simulink model "block_model2018a"  (R2018a)
settings: Solver=VariableStepAuto  StartTime=0.0  StopTime=80  RelTol=1e-3
undefined symbols (not defined in the file or in its folder): DiscIntNeverNeededParam
libraries: simulink x4
settings Model: Creator=igorbeduin  LastModifiedBy=igorbeduin
settings DataIOCC: ReturnWorkspaceOutputs=on
settings SFSimCC: SimUseLocalCustomCode=on
settings RTWCC: RTWUseLocalCustomCode=on

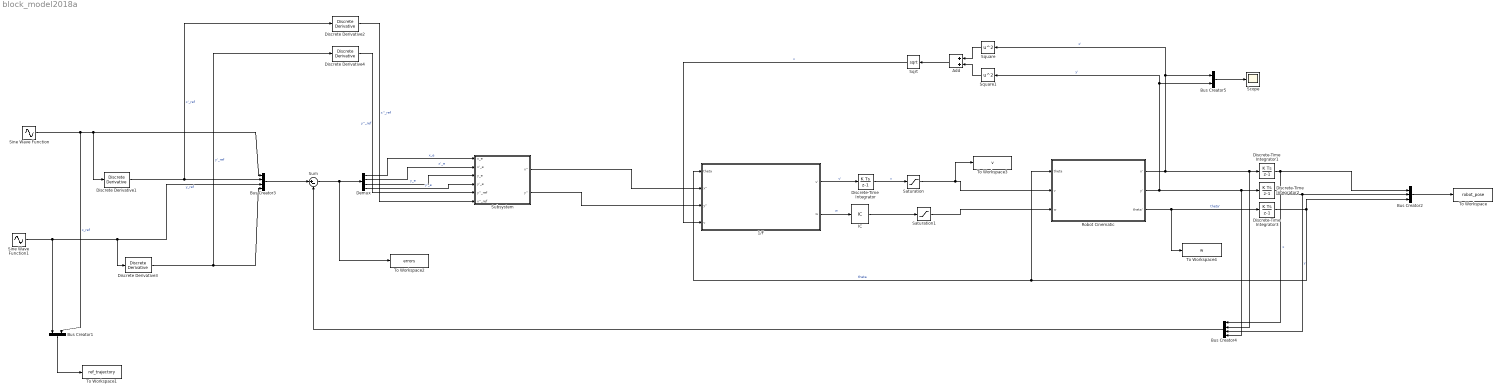
== system block_model2018a ==
  1/F : Subsystem
  Add : Sum
  Bus Creator1 : BusCreator  Inputs=2
  Bus Creator2 : BusCreator  Inputs=3
  Bus Creator3 : BusCreator  Inputs=4
  Bus Creator4 : BusCreator  Inputs=4
  Bus Creator5 : BusCreator  Inputs=2
  Demux : Demux
  Discrete Derivative{1..4} (4 alike) : simulink/Discrete/Discrete Derivative  gainval=1.0  ICPrevScaledInput=0  OutMin=[]  OutMax=[]  OutDataType=fixdt(1, 16)  OutScaling=2^-10  DoSatur=off
  Discrete-Time Integrator : DiscreteIntegrator  SampleTime=0.016  ICPrevOutput=DiscIntNeverNeededParam  ICPrevScaledInput=DiscIntNeverNeededParam
  Discrete-Time Integrator1 : DiscreteIntegrator  InitialCondition=0.5  SampleTime=-1  ICPrevOutput=DiscIntNeverNeededParam  ICPrevScaledInput=DiscIntNeverNeededParam
  Discrete-Time Integrator2 : DiscreteIntegrator  InitialCondition=-0.5  SampleTime=-1  ICPrevOutput=DiscIntNeverNeededParam  ICPrevScaledInput=DiscIntNeverNeededParam
  Discrete-Time Integrator3 : DiscreteIntegrator  SampleTime=-1  ICPrevOutput=DiscIntNeverNeededParam  ICPrevScaledInput=DiscIntNeverNeededParam
  IC : InitialCondition  Value=0
  Robot Cinematic : Subsystem
  Saturation : Saturate  UpperLimit=1.2  LowerLimit=-1.2
  Saturation1 : Saturate  UpperLimit=40  LowerLimit=-40
  Scope : Scope
  Sine Wave Function : Sin  Frequency=2*pi/30  SampleTime=0.016
  Sine Wave Function1 : Sin  Frequency=2*2*pi/30  SampleTime=0.016
  Sqrt : Sqrt  SaturateOnIntegerOverflow=on
  Square : Math  Operator=square  SaturateOnIntegerOverflow=on
  Square1 : Math  Operator=square  SaturateOnIntegerOverflow=on
  Subsystem : Subsystem
  Sum : Sum  Inputs=|+-
  To Workspace : ToWorkspace  VariableName=robot_pose  SaveFormat=Timeseries  SampleTime=-1
  To Workspace1 : ToWorkspace  VariableName=ref_trajectory  SaveFormat=Timeseries  SampleTime=-1
  To Workspace2 : ToWorkspace  VariableName=errors  SaveFormat=Timeseries  SampleTime=-1
  To Workspace3 : ToWorkspace  VariableName=v  SaveFormat=Timeseries  SampleTime=-1
  To Workspace4 : ToWorkspace  VariableName=w  SaveFormat=Timeseries  SampleTime=-1
  wires:
  Robot Cinematic/1(x') -> Bus Creator4/2, Discrete-Time Integrator1/1, Square/1, Bus Creator5/1  "x'"
  Robot Cinematic/2(y') -> Bus Creator4/4, Discrete-Time Integrator2/1, Bus Creator5/2, Square1/1  "y'"
  Robot Cinematic/3(theta') -> To Workspace4/1, Discrete-Time Integrator3/1  "theta'"
  1/F/1(v') -> Discrete-Time Integrator/1  "v'"
  1/F/2(w) -> IC/1  "w"
  Discrete-Time Integrator1/1 -> Bus Creator2/1, Bus Creator4/1  "x"
  Discrete-Time Integrator2/1 -> Bus Creator2/2, Bus Creator4/3  "y"
  Discrete-Time Integrator3/1 -> Robot Cinematic/1(theta), 1/F/1(theta), Bus Creator2/3  "theta"
  Discrete Derivative1/1 -> Discrete Derivative2/1, Bus Creator3/2  "x'_ref"
  Discrete Derivative3/1 -> Bus Creator3/4, Discrete Derivative4/1  "y'_ref"
  Discrete Derivative2/1 -> Subsystem/6(x''_ref)  "x''_ref"
  Discrete Derivative4/1 -> Subsystem/5(y''_ref)  "y''_ref"
  Subsystem/1(x'') -> 1/F/2(x'')
  Subsystem/2(y'') -> 1/F/3(y'')
  Square/1 -> Add/1
  Square1/1 -> Add/2
  Add/1 -> Sqrt/1
  Sqrt/1 -> 1/F/4(v)  "v"
  Bus Creator2/1 -> To Workspace/1
  Bus Creator1/1 -> To Workspace1/1
  Bus Creator3/1 -> Sum/1
  Bus Creator4/1 -> Sum/2
  Sum/1 -> To Workspace2/1, Demux/1
  Demux/1 -> Subsystem/1(x_e)  "x_e"
  Demux/2 -> Subsystem/2(x'_e)  "x'_e"
  Demux/3 -> Subsystem/3(y_e)  "y_e"
  Demux/4 -> Subsystem/4(y'_e)  "y'_e"
  Discrete-Time Integrator/1 -> Saturation/1  "v"
  Bus Creator5/1 -> Scope/1
  Saturation/1 -> To Workspace3/1, Robot Cinematic/2(v)
  Saturation1/1 -> Robot Cinematic/3(w)
  IC/1 -> Saturation1/1
  Sine Wave Function/1 -> Bus Creator3/1, Discrete Derivative1/1, Bus Creator1/2  "x_ref"
  Sine Wave Function1/1 -> Bus Creator3/3, Discrete Derivative3/1, Bus Creator1/1  "y_ref"

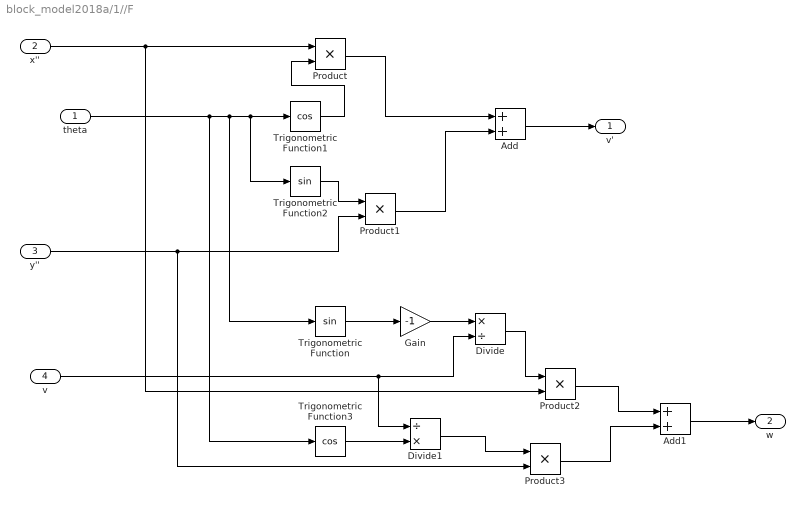
== system block_model2018a/1//F ==
  theta : Inport
  x'' : Inport  Port=2
  y'' : Inport  Port=3
  v : Inport  Port=4
  Add : Sum
  Add1 : Sum
  Divide : Product  Inputs=*/
  Divide1 : Product  Inputs=/*
  Gain : Gain  Gain=-1
  Product{,1..3} (4 alike) : Product
  Trigonometric Function : Trigonometry
  Trigonometric Function1 : Trigonometry  Operator=cos
  Trigonometric Function2 : Trigonometry
  Trigonometric Function3 : Trigonometry  Operator=cos
  v' : Outport
  w : Outport  Port=2
  wires:
  x''/1 -> Product2/2, Product/1
  theta/1 -> Trigonometric Function/1, Trigonometric Function2/1, Trigonometric Function1/1, Trigonometric Function3/1
  Trigonometric Function1/1 -> Product/2
  Product/1 -> Add/1
  Trigonometric Function2/1 -> Product1/1
  y''/1 -> Product3/2, Product1/2
  Product1/1 -> Add/2
  Add/1 -> v'/1
  Trigonometric Function/1 -> Gain/1
  Gain/1 -> Divide/1
  v/1 -> Divide1/1, Divide/2
  Divide/1 -> Product2/1
  Product2/1 -> Add1/1
  Trigonometric Function3/1 -> Divide1/2
  Divide1/1 -> Product3/1
  Product3/1 -> Add1/2
  Add1/1 -> w/1

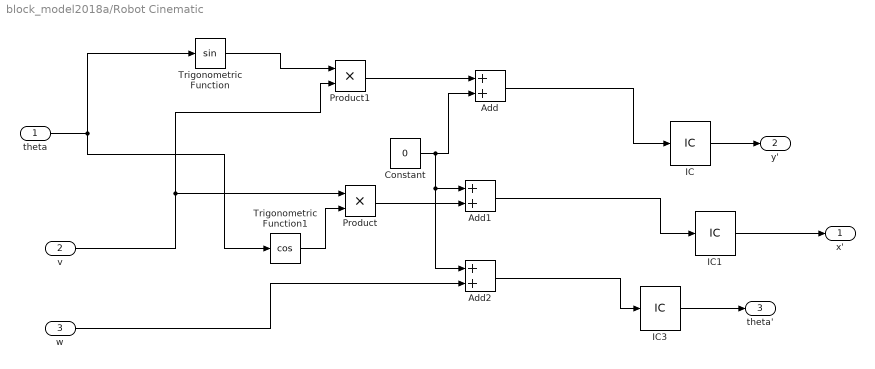
== system block_model2018a/Robot Cinematic ==
  theta : Inport
  v : Inport  Port=2
  w : Inport  Port=3
  Add : Sum
  Add1 : Sum
  Add2 : Sum
  Constant : Constant  Value=0
  IC : InitialCondition  Value=0.5
  IC1 : InitialCondition  Value=0.5
  IC3 : InitialCondition  Value=0
  Product : Product
  Product1 : Product
  Trigonometric Function : Trigonometry
  Trigonometric Function1 : Trigonometry  Operator=cos
  x' : Outport
  y' : Outport  Port=2
  theta' : Outport  Port=3
  wires:
  theta/1 -> Trigonometric Function1/1, Trigonometric Function/1
  Trigonometric Function/1 -> Product1/1
  v/1 -> Product1/2, Product/1
  Trigonometric Function1/1 -> Product/2
  Product1/1 -> Add/1
  Constant/1 -> Add2/1, Add1/1, Add/2
  Product/1 -> Add1/2
  w/1 -> Add2/2
  Add1/1 -> IC1/1
  Add/1 -> IC/1
  IC/1 -> y'/1
  IC1/1 -> x'/1
  Add2/1 -> IC3/1
  IC3/1 -> theta'/1

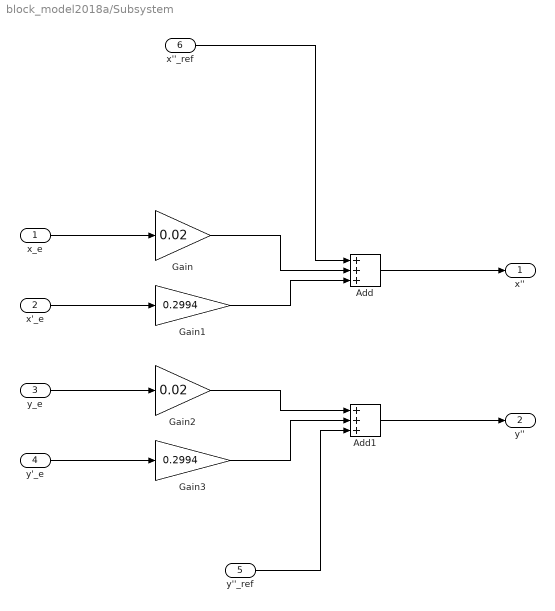
== system block_model2018a/Subsystem ==
  x_e : Inport
  x'_e : Inport  Port=2
  y_e : Inport  Port=3
  y'_e : Inport  Port=4
  y''_ref : Inport  Port=5
  x''_ref : Inport  Port=6
  Add : Sum  Inputs=+++
  Add1 : Sum  Inputs=+++
  Gain : Gain  Gain=0.02
  Gain1 : Gain  Gain=0.2994
  Gain2 : Gain  Gain=0.02
  Gain3 : Gain  Gain=0.2994
  x'' : Outport
  y'' : Outport  Port=2
  wires:
  x_e/1 -> Gain/1
  x'_e/1 -> Gain1/1
  Add/1 -> x''/1
  y_e/1 -> Gain2/1
  y'_e/1 -> Gain3/1
  Add1/1 -> y''/1
  Gain1/1 -> Add/3
  Gain/1 -> Add/2
  x''_ref/1 -> Add/1
  y''_ref/1 -> Add1/3
  Gain2/1 -> Add1/1
  Gain3/1 -> Add1/2
